simulink model "modeleAvion"  (R2019a)
settings: Solver=ode45  StartTime=0.0  StopTime=60.0  RelTol=1e-3  EnableMultiTasking=on
values from neighbouring files (symbols this model uses):
  DEG2RAD = pi/180    (= 0.0174532925199)    [startCADV.m]    (also in stcr.m)
  g = 9.80665    [startCADV.m]
  gammae = 0*DEG2RAD    (= 0)    [startCADV.m]
  k = KTS2MS /(2*FL2M)    (= 0.00843904928551)    [startCADV.m]
  k11 = 0.1    [startCADV.m]
  k22 = 1    [startCADV.m]
  KTS2MS = NM2M / 3600    (= 0.514444444444)    [startCADV.m]
  phie = 0*5*DEG2RAD    (= 0)    [startCADV.m]
  psie = 0*DEG2RAD    (= 0)    [startCADV.m]
  Ve = Vie + k*ze    (= 66.8777777778)    [startCADV.m]
  Vie = 130*KTS2MS    (= 66.8777777778)    [startCADV.m]
  ze = 0*100*FL2M    (= 0)    [startCADV.m]
settings Model: Creator=thierry  LastModifiedBy=silvabjo
settings DataIOCC: LimitDataPoints=on  SaveFormat=Array  ReturnWorkspaceOutputs=off
settings OptimizationCC: LifeSpan=inf
settings DebuggingCC: UnderspecifiedInitializationDetection=Classic  MergeDetectMultiDrivingBlocksExec=none  StateNameClashWarn=warning  SFUnexpectedBacktrackingDiag=warning  SFNoUnconditionalDefaultTransitionDiag=warning  SFExecutionAtInitializationDiag=none  ArithmeticOperatorsInVariantConditions=warning
settings HardwareCC: ProdBitPerPointer=32  ProdBitPerSizeT=32  ProdBitPerPtrDiffT=32  ProdLargestAtomicFloat=None  ProdIntDivRoundTo=Undefined  ProdEndianess=Unspecified  ProdWordSize=32  ProdHWDeviceType=32-bit Generic
settings ModelReferenceCC: PropagateSignalLabelsOutOfModel=off
settings SFSimCC: SimUseLocalCustomCode=off
settings RTWCC: RTWUseLocalCustomCode=off
settings CodeAppCC: StateflowObjectComments=on
settings GRTTargetCC: TargetLangStandard=C89/C90 (ANSI)
settings ConfigComp: CovMetricSettings=dw  CovSaveCumulativeToWorkspaceVar=on  CovSaveSingleToWorkspaceVar=on  CovExternalEMLEnable=off

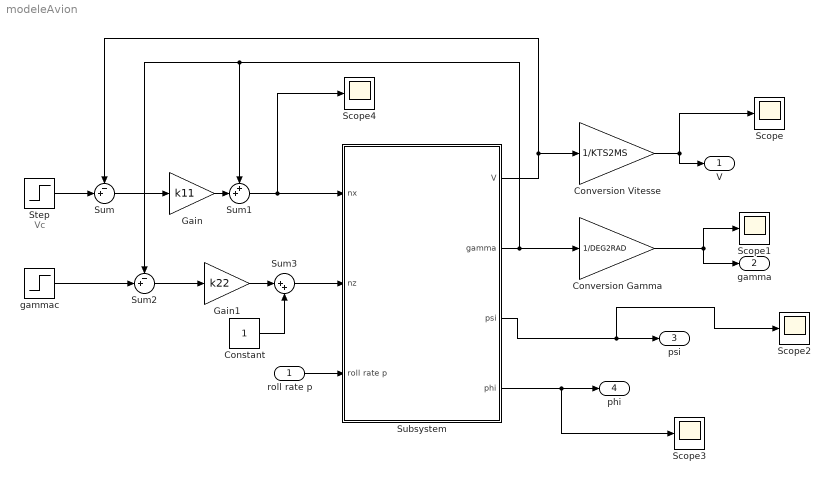
== system modeleAvion ==
  note: Vc
  roll rate p : Inport
  Constant : Constant
  Conversion Gamma : Gain  Gain=1/DEG2RAD
  Conversion Vitesse : Gain  Gain=1/KTS2MS
  Gain : Gain  Gain=k11
  Gain1 : Gain  Gain=k22
  Scope{,1..4} (5 alike) : Scope
  Step : Step  Before=Ve  After=Ve  SampleTime=0
  Subsystem : Subsystem
  Sum : Sum  Inputs=-+|
  Sum1 : Sum  Inputs=++|
  Sum2 : Sum  Inputs=-+|
  Sum3 : Sum  Inputs=|++
  "gammac " : Step  Time=10  After=3*DEG2RAD  SampleTime=0
  V : Outport
  gamma : Outport  Port=2
  psi : Outport  Port=3
  phi : Outport  Port=4
  wires:
  Sum1/1 -> Scope4/1, Subsystem/1(nx)
  Gain1/1 -> Sum3/1
  roll rate p/1 -> Subsystem/3(roll rate p)
  Subsystem/1(V) -> Sum/1, Conversion Vitesse/1
  Subsystem/2(gamma) -> Sum2/1, Sum1/1, Conversion Gamma/1
  Subsystem/3(psi) -> Scope2/1, psi/1
  Subsystem/4(phi) -> Scope3/1, phi/1
  Gain/1 -> Sum1/2
  Sum/1 -> Gain/1
  Step/1 -> Sum/2
  "gammac "/1 -> Sum2/2
  Sum2/1 -> Gain1/1
  Sum3/1 -> Subsystem/2(nz)
  Constant/1 -> Sum3/2
  Conversion Vitesse/1 -> V/1, Scope/1
  Conversion Gamma/1 -> Scope1/1, gamma/1

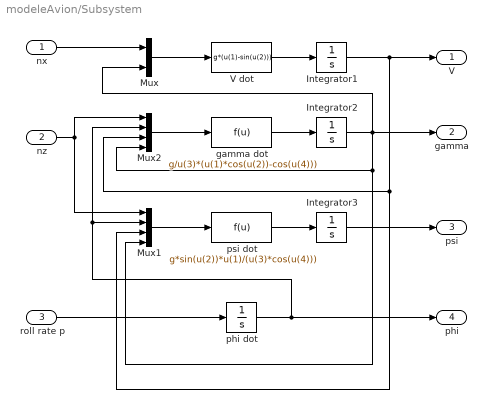
== system modeleAvion/Subsystem ==
  nx : Inport
  nz : Inport  Port=2
  roll rate p : Inport  Port=3
  Integrator1 : Integrator  InitialCondition=Vie + k*ze
  Integrator2 : Integrator  InitialCondition=gammae
  Integrator3 : Integrator  InitialCondition=psie
  Mux : Mux  Inputs=2
  Mux1 : Mux
  Mux2 : Mux
  V dot : Fcn  Expr=g*(u(1)-sin(u(2)))
  gamma dot : Fcn  Expr=g/u(3)*(u(1)*cos(u(2))-cos(u(4)))
  phi dot : Integrator  InitialCondition=phie
  psi dot : Fcn  Expr=g*sin(u(2))*u(1)/(u(3)*cos(u(4)))
  V : Outport
  gamma : Outport  Port=2
  psi : Outport  Port=3
  phi : Outport  Port=4
  wires:
  roll rate p/1 -> phi dot/1
  nx/1 -> Mux/1
  nz/1 -> Mux1/1, Mux2/1
  Mux2/1 -> gamma dot/1
  phi dot/1 -> phi/1, Mux1/2, Mux2/2
  Mux/1 -> V dot/1
  psi dot/1 -> Integrator3/1
  Integrator3/1 -> psi/1
  Mux1/1 -> psi dot/1
  gamma dot/1 -> Integrator2/1
  Integrator1/1 -> V/1, Mux2/3, Mux1/3
  V dot/1 -> Integrator1/1
  Integrator2/1 -> gamma/1, Mux/2, Mux2/4, Mux1/4
